simulink library "lib_Engine"  (R2017b)
settings: Solver=VariableStepAuto  StartTime=0.0  StopTime=10.0  RelTol=1e-3
undefined symbols (not defined in the file): air, Engine, env, max_vehicle_rad_air_flow
libraries: Pneumatic_lib x11, nesl_utility x9, simulink x5, EC2_libraries x1, fl_lib x1
settings Model: Creator=Di Russo  LastModifiedBy=Lyu19
settings CodeAppCC: StateflowObjectComments=on

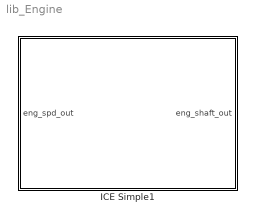
== system lib_Engine ==
  ICE Simple1 : Subsystem
      mask Display:
      | image(imread('EngineTopLevel.jpg'),'center')
      | color('red');
      | port_label('input',1,'SpdOut')
      | port_label('output',1,'ShaftOut')

== system lib_Engine/ICE Simple1 ==
  eng_spd_out : Inport
  Engine Plant Modified : Subsystem
      mask Display:
      | image(imread('EngineTopLevel.jpg'),'center')
      | color('red');
      | port_label('input',2,'SpdOut')
      | port_label('output',2,'ShaftOut')
  Inputs : Subsystem
  Soft ECM : Subsystem
      mask Display: image('SoftECU.jpg')
  eng_shaft_out : Outport
  tag scope: ECM_to_HCU=global
  wires:
  Engine Plant Modified/1(Out) -> Soft ECM/2(In1)
  Soft ECM/1(Out) -> [ECM_to_HCU]
  Inputs/1(Inputs) -> Soft ECM/1(In)
  Soft ECM/2(Out1) -> Engine Plant Modified/1("In ")  "ECM_to_Actuators"
  eng_spd_out/1 -> Engine Plant Modified/2(eng_spd_out)
  Engine Plant Modified/2(eng_shaft_out) -> eng_shaft_out/1

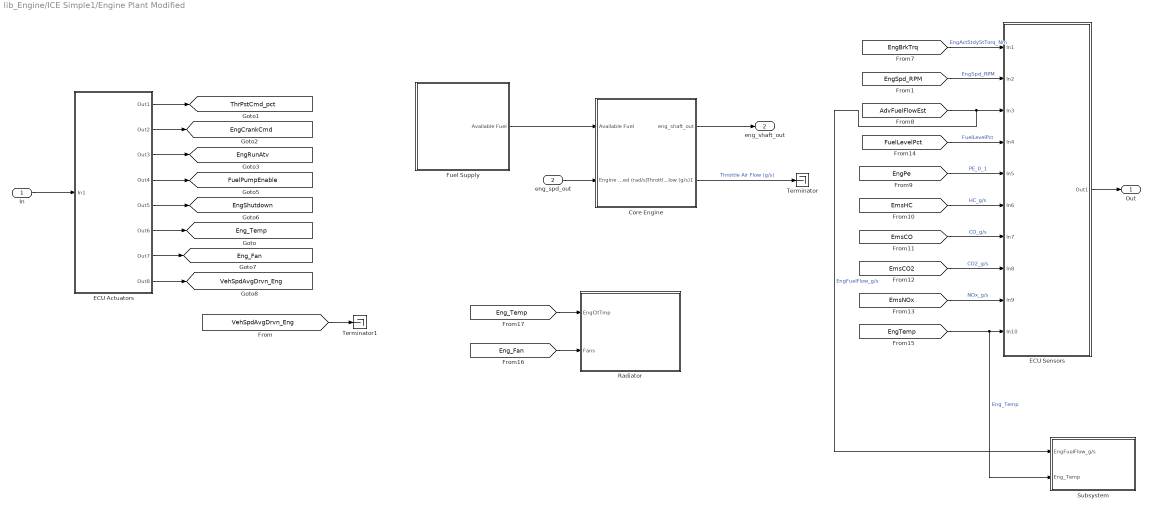
== system lib_Engine/ICE Simple1/Engine Plant Modified ==
  "In " : Inport
  eng_spd_out : Inport  Port=2
  Core Engine : Subsystem
      mask Display: image(imread('EngineShortBlock.jpg'),'center')
  ECU Actuators : Subsystem
  ECU Sensors : Subsystem
  Fuel Supply : Subsystem
      mask Display: image(imread('FuelTank.jpg'),'center')
  Radiator : Subsystem
  Subsystem : Subsystem
  Terminator : Terminator
  Terminator1 : Terminator
  Out : Outport
  eng_shaft_out : Outport  Port=2
  tag scope: EngCrankCmd=global, EngRunAtv=global, EngShutdown=global, Eng_Fan=global, Eng_Temp=global, FuelPumpEnable=global, ThrPstCmd_pct=global, VehSpdAvgDrvn_Eng=global
  wires:
  [VehSpdAvgDrvn_Eng] -> Terminator1/1
  Core Engine/2(Throttle Air Flow (g/s)1) -> Terminator/1  "Throttle Air Flow (g/s)"
  ECU Sensors/1(Out1) -> Out/1
  ECU Actuators/8(Out8) -> [VehSpdAvgDrvn_Eng]
  ECU Actuators/7(Out7) -> [Eng_Fan]
  ECU Actuators/6(Out6) -> [Eng_Temp]
  [Eng_Temp] -> Radiator/1(EngCltTmp)
  [Eng_Fan] -> Radiator/2(Fans)
  eng_spd_out/1 -> Core Engine/2(Engine Speed (rad/s))
  Core Engine/1(eng_shaft_out) -> eng_shaft_out/1
  ECU Actuators/3(Out3) -> [EngRunAtv]
  ECU Actuators/2(Out2) -> [EngCrankCmd]
  [EngSpd_RPM] -> ECU Sensors/2(In2)  "EngSpd_RPM"
  [EngBrkTrq] -> ECU Sensors/1(In1)  "EngActStdyStTorq_Nm"
  "In "/1 -> ECU Actuators/1(In1)
  ECU Actuators/1(Out1) -> [ThrPstCmd_pct]
  ECU Actuators/4(Out4) -> [FuelPumpEnable]
  Fuel Supply/1(Available Fuel) -> Core Engine/1(Available Fuel)
  [EmsNOx] -> ECU Sensors/9(In9)  "NOx_g/s"
  [EmsCO2] -> ECU Sensors/8(In8)  "CO2_g/s"
  [EmsCO] -> ECU Sensors/7(In7)  "CO_g/s"
  [EngPe] -> ECU Sensors/5(In5)  "PE_0_1"
  [EmsHC] -> ECU Sensors/6(In6)  "HC_g/s"
  [FuelLevelPct] -> ECU Sensors/4(In4)  "FuelLevelPct"
  ECU Actuators/5(Out5) -> [EngShutdown]
  [EngTemp] -> ECU Sensors/10(In10), Subsystem/2(Eng_Temp)  "Eng_Temp"
  [AdvFuelFlowEst] -> Subsystem/1(EngFuelFlow_g/s), ECU Sensors/3(In3)  "EngFuelFlow_g/s"

== system lib_Engine/ICE Simple1/Inputs ==
  Analog : Subsystem
  Bus Creator : BusCreator  Inputs=2
  CAN_from_HCU : Subsystem
  Inputs : Outport
  wires:
  Bus Creator/1 -> Inputs/1
  Analog/1(Out1) -> Bus Creator/2  "Analog"
  CAN_from_HCU/1(Out1) -> Bus Creator/1  "CAN"

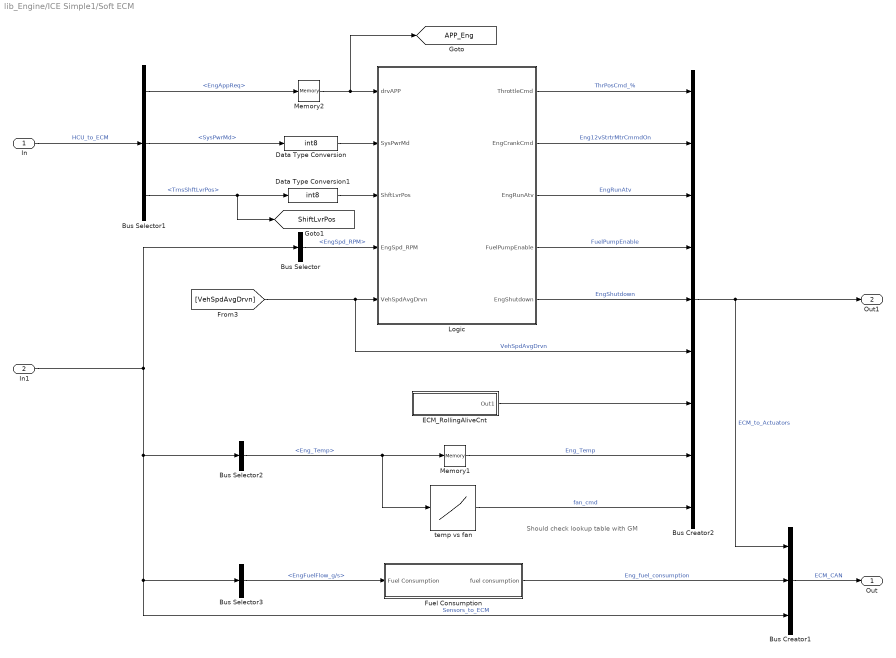
== system lib_Engine/ICE Simple1/Soft ECM ==
  note: Should check lookup table with GM
  In : Inport
  In1 : Inport  Port=2
  Bus Creator1 : BusCreator  Inputs=3
  Bus Creator2 : BusCreator  Inputs=9
  Bus Selector : BusSelector  OutputSignals=EngSpd_RPM
  Bus Selector1 : BusSelector  OutputSignals=Analog.EngAppReq,CAN.to EBCAN.PPEI_Platform_General_Status.SysPwrMd,CAN.to EBCAN.PPEI_Trans_General_Status_2.TrnsShftLvrPos
  Bus Selector2 : BusSelector  OutputSignals=Eng_Temp
  Bus Selector3 : BusSelector  OutputSignals=EngFuelFlow_g/s
  Data Type Conversion : DataTypeConversion  OutDataTypeStr=int8
  Data Type Conversion1 : DataTypeConversion  OutDataTypeStr=int8
  ECM_RollingAliveCnt : Subsystem
  Fuel Consumption : Subsystem
  Logic : Stateflow chart  TreatAsAtomicUnit=on
  Memory1 : Memory  InitialCondition=Engine.Init_T_amb
  Memory2 : Memory
  temp vs fan : Lookup_n-D  NumberOfTableDimensions=1  BreakpointsForDimension1=[0:1:100]  Table=[0:0.01:1]  InternalRulePriority=Speed  RndMeth=Simplest  InputSameDT=on
  Out : Outport
  Out1 : Outport  Port=2
  tag scope: APP_Eng=global, ShiftLvrPos=global
  wires:
  [VehSpdAvgDrvn] -> Logic/5(VehSpdAvgDrvn), Bus Creator2/6  "VehSpdAvgDrvn"
  In/1 -> Bus Selector1/1  "HCU_to_ECM"
  Memory2/1 -> Logic/1(drvAPP), [APP_Eng]
  Data Type Conversion1/1 -> Logic/3(ShftLvrPos)
  Data Type Conversion/1 -> Logic/2(SysPwrMd)
  ECM_RollingAliveCnt/1(Out1) -> Bus Creator2/7
  Memory1/1 -> Bus Creator2/8  "Eng_Temp"
  temp vs fan/1 -> Bus Creator2/9  "fan_cmd"
  Fuel Consumption/1(fuel consumption) -> Bus Creator1/2  "Eng_fuel_consumption"
  Bus Selector3/1 -> Fuel Consumption/1(Fuel Consumption)  "<EngFuelFlow_g/s>"
  Bus Selector2/1 -> Memory1/1, temp vs fan/1  "<Eng_Temp>"
  Logic/5(EngShutdown) -> Bus Creator2/5  "EngShutdown"
  Bus Selector1/3 -> Data Type Conversion1/1, [ShiftLvrPos]  "<TrnsShftLvrPos>"
  Bus Selector1/2 -> Data Type Conversion/1  "<SysPwrMd>"
  Logic/4(FuelPumpEnable) -> Bus Creator2/4  "FuelPumpEnable"
  In1/1 -> Bus Selector/1, Bus Selector2/1, Bus Selector3/1, Bus Creator1/3  "Sensors_to_ECM"
  Logic/1(ThrottleCmd) -> Bus Creator2/1  "ThrPosCmd_%"
  Bus Creator2/1 -> Bus Creator1/1, Out1/1  "ECM_to_Actuators"
  Bus Creator1/1 -> Out/1  "ECM_CAN"
  Logic/2(EngCrankCmd) -> Bus Creator2/2  "Eng12vStrtrMtrCmmdOn"
  Bus Selector1/1 -> Memory2/1  "<EngAppReq>"
  Bus Selector/1 -> Logic/4(EngSpd_RPM)  "<EngSpd_RPM>"
  Logic/3(EngRunAtv) -> Bus Creator2/3  "EngRunAtv"

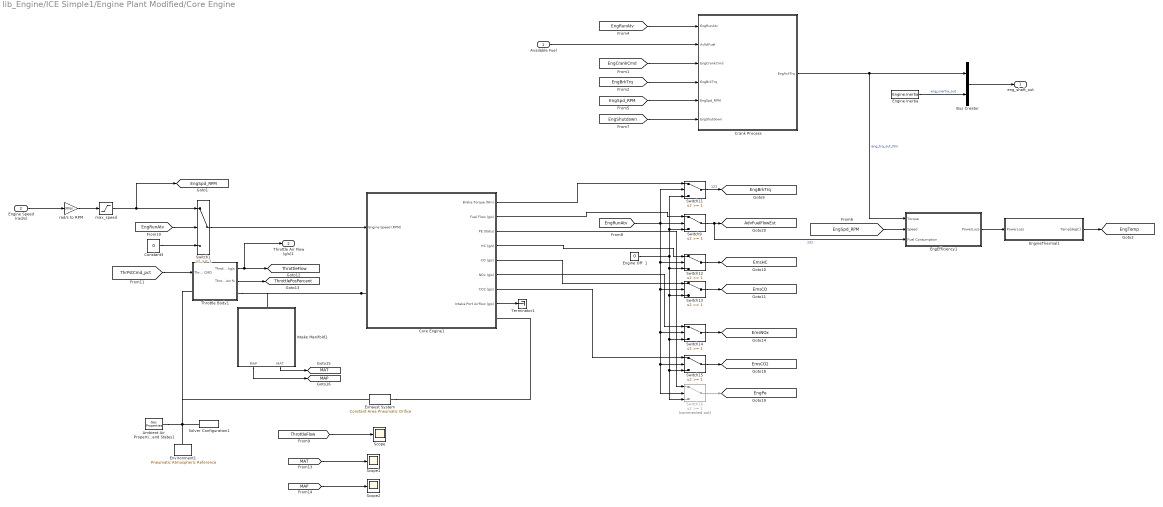
== system lib_Engine/ICE Simple1/Engine Plant Modified/Core Engine ==
  Available Fuel : Inport
  Engine Speed (rad/s) : Inport  Port=2
  Ambient Air Properties and States1 : Pneumatic_lib/Pneumatic Utilities/Gas Properties  c_p=1.005e+3 J/kg/K  c_v=717.95 J/kg/K  viscosity=1.821e-5 s*Pa  Pa=100 kPa  Ta=293.15 K  range_error=1
  Bus Creator : BusCreator  Inputs=2
  Constant3 : Constant  Value=0
  Core Engine1 : Subsystem
      mask Display: image(imread('EngineShortBlock.jpg'),'center')
  Crank Process : Stateflow chart  TreatAsAtomicUnit=on
  EngEfficiency1 : Subsystem
  Engine Inertia : Constant  Value=Engine.Inertia
  Engine Off  1 : Constant  Value=0
  EngineThermal1 : Subsystem
  Environment1 : Pneumatic_lib/Pneumatic Elements/Pneumatic Atmospheric Reference
  Exhaust System : Pneumatic_lib/Pneumatic Elements/Constant Area Pneumatic Orifice  Cd=0.8  Area=0.25*pi*(4*0.0254)^2 m^2  G_specify=off  G_priority=High  G=0 kg/s  G_nominal_specify=off  G_nominal_unit=kg/s  G_nominal_value=1  Q1_specify=off  Q1_priority=High  Q1=0 J/s  Q1_nominal_specify=off  Q1_nominal_unit=J/s  Q1_nominal_value=1  Q2_specify=off  Q2_priority=High  Q2=0 J/s  Q2_nominal_specify=off  Q2_nominal_unit=J/s  Q2_nominal_value=1  p1_specify=off  p1_priority=High  p1=1e+5 Pa  p1_nominal_specify=off  p1_nominal_unit=Pa  p1_nominal_value=1  p2_specify=off  p2_priority=High  p2=1e+5 Pa  p2_nominal_specify=off  p2_nominal_unit=Pa  p2_nominal_value=1  T1_specify=off  T1_priority=High  T1=300 K  T1_nominal_specify=off  T1_nominal_unit=K  T1_nominal_value=1  T2_specify=off  T2_priority=High  T2=300 K  T2_nominal_specify=off  T2_nominal_unit=K  T2_nominal_value=1
  Intake Manifold1 : Subsystem
      mask Display: image(imread('IntakeManifold.jpg'),'center')
  Scope : Scope
  Scope1 : Scope
  Scope2 : Scope
  Solver Configuration1 : nesl_utility/Solver Configuration  PhysicalDomain=network_engine_domain  SubClassName=solver  LeftPortType=input  RightPortType=generic  Accelerate=off  Tones=[]  Harmonics=[]  SimulateNoise=off  Profile=off  UseLocalSampling=off  EnableSwitchedLinearOptims=on  FrequencyDomain=off  UseCCode=off  RelTol=0.001  AbsTol=1e-06  MinStep=1e-09  ToWorkspace=off  RevertToSquareIcSolve=off  NumHomotopyIterations=100  PhasorMode=off  PhasorModeNumHarmonics=1  DoDC=off  ResidualTolerance=1e-9  UseLocalSolver=on  LocalSolverChoice=NE_BACKWARD_EULER_ADVANCER  LocalSolverSampleTime=.01  DoFixedCost=off  MaxNonlinIter=3  MaxModeIter=2  LinearAlgebra=Sparse  DelaysMemoryBudget=1024  AutomaticFiltering=on  FilteringTimeConstant=0.001
  Switch{1,9,11..15} (7 alike) : Switch  Threshold=1
  Switch16 : Switch  Commented=on  Threshold=1
  Terminator1 : Terminator
  Throttle Body1 : Subsystem
      mask Display: image(imread('ElectronicThrottle.jpg'),'center')
  max_speed : Saturate  UpperLimit=max(Engine.Engine.TQ.SPEED)  LowerLimit=0
  rad/s to RPM : Gain  Gain=30/pi
  eng_shaft_out : Outport
  Throttle Air Flow (g/s)1 : Outport  Port=2
  tag scope: AdvFuelFlowEst=global, EmsCO2=global, EmsCO=global, EmsHC=global, EmsNOx=global, EngBrkTrq=global, EngPe=global, EngSpd_RPM=global, EngTemp=global, MAP=global, MAT=global, ThrottleFlow=global, ThrottlePosPercent=global
  wires:
  Engine Speed (rad/s)/1 -> rad/s to RPM/1
  max_speed/1 -> Switch1/1, [EngSpd_RPM]
  rad/s to RPM/1 -> max_speed/1
  [MAP] -> Scope2/1
  [MAT] -> Scope1/1
  [ThrottleFlow] -> Scope/1
  [EngBrkTrq] -> Crank Process/4(EngBrkTrq)
  [EngShutdown] -> Crank Process/6(EngShutdown)
  [EngRunAtv] -> Crank Process/1(EngRunAtv)
  Bus Creator/1 -> eng_shaft_out/1
  Available Fuel/1 -> Crank Process/2(AvlblFuel)
  [EngCrankCmd] -> Crank Process/3(EngCrankCmd)
  [EngSpd_RPM] -> Crank Process/5(EngSpd_RPM)
  Engine Inertia/1 -> Bus Creator/2  "eng_inertia_out"
  Engine Off  1/1 -> Switch12/3, Switch13/3, Switch14/3, Switch15/3, Switch16/3, Switch11/3, Switch9/3
  Core Engine1/5(CO (g/s)) -> Switch13/1
  Core Engine1/2(Fuel Flow (g/s)) -> Switch9/1
  Core Engine1/7(CO2 (g/s)) -> Switch15/1
  Switch12/1 -> [EmsHC]
  Switch11/1 -> [EngBrkTrq]  "123"
  Switch15/1 -> [EmsCO2]
  Switch9/1 -> EngEfficiency1/3(Fuel Consumption), [AdvFuelFlowEst]  "131"
  [EngSpd_RPM] -> EngEfficiency1/2(Speed)
  Switch13/1 -> [EmsCO]
  EngineThermal1/1(Temp[degC]) -> [EngTemp]
  Core Engine1/6(NOx (g/s)) -> Switch14/1
  Switch14/1 -> [EmsNOx]
  [EngRunAtv] -> Switch9/2, Switch12/2, Switch15/2, Switch16/2, Switch14/2, Switch13/2, Switch11/2
  EngEfficiency1/1(PowerLoss) -> EngineThermal1/1(PowerLoss)
  Crank Process/1(EngActTrq) -> Bus Creator/1, EngEfficiency1/1(Torque)  "eng_trq_out_Nm"
  Switch16/1 -> [EngPe]
  Core Engine1/1(Brake Torque (Nm)) -> Switch11/1
  Core Engine1/4(HC (g/s)) -> Switch12/1
  Core Engine1/3(PE Status) -> Switch16/1
  [ThrPstCmd_pct] -> Throttle Body1/1(Throttle Position % CMD)
  Switch1/1 -> Core Engine1/1(Engine Speed (RPM))
  Constant3/1 -> Switch1/3
  [EngRunAtv] -> Switch1/2
  Throttle Body1/1(Throttle Flow kg/s) -> [ThrottleFlow], Throttle Air Flow (g/s)1/1
  Intake Manifold1/2(MAT) -> [MAT]
  Intake Manifold1/1(MAP) -> [MAP]
  Core Engine1/8(Intake Port Airflow (g/s)) -> Terminator1/1
  Throttle Body1/2(Throttle Position %) -> [ThrottlePosPercent]
  connections:
  Exhaust System/LConn1 -- Core Engine1/RConn1
  Core Engine1/LConn1 -- Intake Manifold1/LConn1 -- Throttle Body1/RConn1
  Ambient Air Properties and States1/RConn1 -- Throttle Body1/LConn1 -- Exhaust System/RConn1 -- Solver Configuration1/RConn1 -- Environment1/LConn1

== system lib_Engine/ICE Simple1/Engine Plant Modified/ECU Actuators ==
  In1 : Inport
  Bus Selector : BusSelector  OutputSignals=ThrPosCmd_%,Eng12vStrtrMtrCmmdOn,EngRunAtv,FuelPumpEnable,EngShutdown,Eng_Temp,fan_cmd,VehSpdAvgDrvn
  Out1 : Outport
  Out2 : Outport  Port=2
  Out3 : Outport  Port=3
  Out4 : Outport  Port=4
  Out5 : Outport  Port=5
  Out6 : Outport  Port=6
  Out7 : Outport  Port=7
  Out8 : Outport  Port=8
  wires:
  Bus Selector/8 -> Out8/1  "<VehSpdAvgDrvn>"
  Bus Selector/7 -> Out7/1  "<fan_cmd>"
  Bus Selector/6 -> Out6/1  "<Eng_Temp>"
  Bus Selector/3 -> Out3/1  "<EngRunAtv>"
  Bus Selector/2 -> Out2/1  "<Eng12vStrtrMtrCmmdOn>"
  Bus Selector/1 -> Out1/1  "<ThrPosCmd_%>"
  In1/1 -> Bus Selector/1
  Bus Selector/4 -> Out4/1  "<FuelPumpEnable>"
  Bus Selector/5 -> Out5/1  "<EngShutdown>"

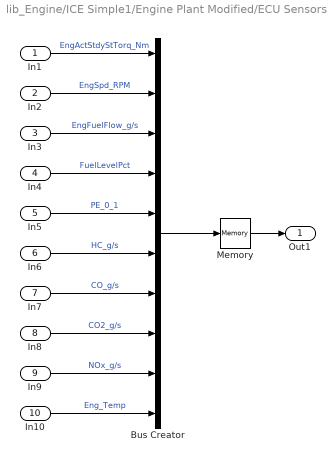
== system lib_Engine/ICE Simple1/Engine Plant Modified/ECU Sensors ==
  In1 : Inport
  In2 : Inport  Port=2
  In3 : Inport  Port=3
  In4 : Inport  Port=4
  In5 : Inport  Port=5
  In6 : Inport  Port=6
  In7 : Inport  Port=7
  In8 : Inport  Port=8
  In9 : Inport  Port=9
  In10 : Inport  Port=10
  Bus Creator : BusCreator  Inputs=10
  Memory : Memory
  Out1 : Outport
  wires:
  Memory/1 -> Out1/1
  In10/1 -> Bus Creator/10  "Eng_Temp"
  In8/1 -> Bus Creator/8  "CO2_g/s"
  Bus Creator/1 -> Memory/1
  In7/1 -> Bus Creator/7  "CO_g/s"
  In6/1 -> Bus Creator/6  "HC_g/s"
  In5/1 -> Bus Creator/5  "PE_0_1"
  In4/1 -> Bus Creator/4  "FuelLevelPct"
  In3/1 -> Bus Creator/3  "EngFuelFlow_g/s"
  In2/1 -> Bus Creator/2  "EngSpd_RPM"
  In1/1 -> Bus Creator/1  "EngActStdyStTorq_Nm"
  In9/1 -> Bus Creator/9  "NOx_g/s"

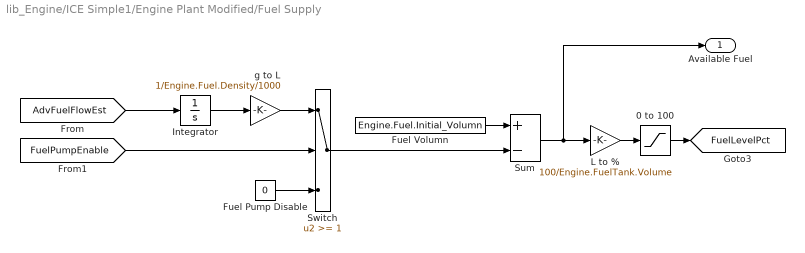
== system lib_Engine/ICE Simple1/Engine Plant Modified/Fuel Supply ==
  0 to 100 : Saturate
  Fuel Pump Disable : Constant  Value=0
  Fuel Volumn : Constant  Value=Engine.Fuel.Initial_Volumn
  Integrator : Integrator  LimitOutput=on  UpperSaturationLimit=Engine.FuelTank.Volume  LowerSaturationLimit=0
  L to % : Gain  Gain=100/Engine.FuelTank.Volume
  Sum : Sum  Inputs=+-
  Switch : Switch  Threshold=1
  g to L : Gain  Gain=1/Engine.Fuel.Density/1000
  Available Fuel : Outport
  tag scope: FuelLevelPct=global
  wires:
  Fuel Volumn/1 -> Sum/1
  Switch/1 -> Sum/2
  Sum/1 -> Available Fuel/1, L to %/1
  [FuelPumpEnable] -> Switch/2
  [AdvFuelFlowEst] -> Integrator/1
  Integrator/1 -> g to L/1
  g to L/1 -> Switch/1
  Fuel Pump Disable/1 -> Switch/3
  L to %/1 -> 0 to 100/1
  0 to 100/1 -> [FuelLevelPct]

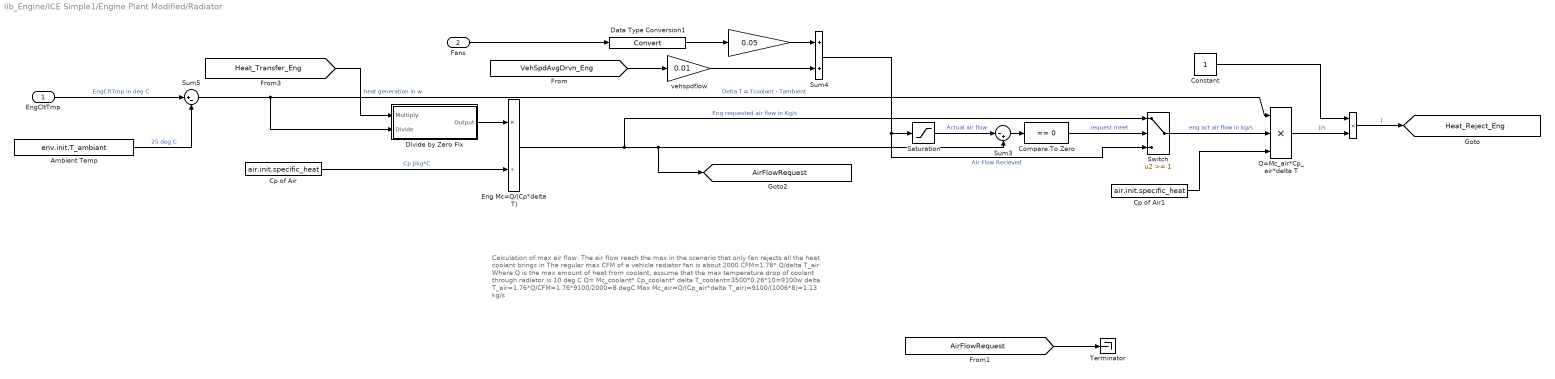
== system lib_Engine/ICE Simple1/Engine Plant Modified/Radiator ==
  note: Calculation of max air flow:
      |
      | The air flow reach the max in the scenario that only fan rejects all the heat coolant brings in
      |
      | The regular max CFM of a vehicle radiator fan is about 2000
      |
      | CFM=1.76* Q/delta T_air
      |
      | Where Q is the max amount of heat from coolant, assume that the max temperature drop of coolant
      | through radiator is 10 deg C
      |
      | Q= Mc_coolant* Cp_coolant* delta T_coolant=3500*0.26*10=9100w
      |
      | delta T_air=1.76*Q/CFM=1.76*9100/2000=8 degC
      |
      | Max Mc_air=Q/(Cp_air*delta T_air)=9100/(1006*8)=1.13 kg/s
  EngCltTmp : Inport
  Fans : Inport  Port=2
  " " : Product  Inputs=**
  " " : Gain  Gain=0.05
  Ambient Temp : Constant  Value=env.init.T_ambiant
  Compare To Zero : simulink/Logic and Bit Operations/Compare To Zero  relop===  OutDataTypeStr=uint8
  Constant : Constant
  Cp of Air : Constant  Value=air.init.specific_heat
  Cp of Air1 : Constant  Value=air.init.specific_heat
  Data Type Conversion1 : DataTypeConversion
  Divide by Zero Fix : Subsystem
  "Eng Mc=Q/(Cp*delta T) " : Product  Inputs=*/
  Q=Mc_air*Cp_air*delta T : Product  Inputs=***
  Saturation : Saturate  UpperLimit=max_vehicle_rad_air_flow  LowerLimit=-1
  Sum3 : Sum  Inputs=|-+
  Sum4 : Sum
  Sum5 : Sum  Inputs=|+-
  Switch : Switch  Threshold=1
  Terminator : Terminator
  vehspdflow : Gain  Gain=0.01
  tag scope: AirFlowRequest=global, Heat_Reject_Eng=global
  wires:
  [AirFlowRequest] -> Terminator/1
  Constant/1 -> " "/1
  " "/1 -> Sum4/1
  Divide by Zero Fix/1(Output) -> "Eng Mc=Q/(Cp*delta T) "/1
  [Heat_Transfer_Eng] -> Divide by Zero Fix/1(Multiply)  "heat generation in w"
  vehspdflow/1 -> Sum4/2
  [VehSpdAvgDrvn_Eng] -> vehspdflow/1
  Fans/1 -> Data Type Conversion1/1
  Sum4/1 -> Saturation/1, Switch/3  "Air Flow Recieved"
  "Eng Mc=Q/(Cp*delta T) "/1 -> [AirFlowRequest], Sum3/2, Switch/1  "Eng requested air flow in Kg/s"
  EngCltTmp/1 -> Sum5/1  "EngCltTmp in deg C"
  Sum5/1 -> Q=Mc_air*Cp_air*delta T/1, Divide by Zero Fix/2(Divide)  "Delta T = Tcoolant - Tambient"
  Ambient Temp/1 -> Sum5/2  "25 deg C"
  Cp of Air/1 -> "Eng Mc=Q/(Cp*delta T) "/2  "Cp J/kg*C"
  Compare To Zero/1 -> Switch/2  "request meet"
  Sum3/1 -> Compare To Zero/1
  Saturation/1 -> Sum3/1  "Actual air flow"
  " "/1 -> [Heat_Reject_Eng]  "J"
  Q=Mc_air*Cp_air*delta T/1 -> " "/2  "J/s"
  Switch/1 -> Q=Mc_air*Cp_air*delta T/2  "eng act air flow in kg/s"
  Cp of Air1/1 -> Q=Mc_air*Cp_air*delta T/3
  Data Type Conversion1/1 -> " "/1

== system lib_Engine/ICE Simple1/Engine Plant Modified/Subsystem ==
  EngFuelFlow_g/s : Inport
  Eng_Temp : Inport  Port=2
  Rate Transition1 : RateTransition  OutPortSampleTime=1
  Rate Transition7 : RateTransition  OutPortSampleTime=1
  To Workspace2 : ToWorkspace  VariableName=EngCltTmp  SampleTime=-1
  To Workspace3 : ToWorkspace  VariableName=InstFuelConsmpRate  SampleTime=-1
  g/s 2 l/hr : Gain  Gain=0.001/0.7871*3600
  wires:
  EngFuelFlow_g/s/1 -> g/s 2 l/hr/1
  Eng_Temp/1 -> Rate Transition1/1
  Rate Transition1/1 -> To Workspace2/1
  g/s 2 l/hr/1 -> Rate Transition7/1
  Rate Transition7/1 -> To Workspace3/1

== system lib_Engine/ICE Simple1/Inputs/Analog ==
  Out1 : Outport
  wires:
  [Analog] -> Out1/1

== system lib_Engine/ICE Simple1/Inputs/CAN_from_HCU ==
  Bus Creator : BusCreator  Inputs=2
  Out1 : Outport
  wires:
  Bus Creator/1 -> Out1/1
  [HCU_to_VEH_CAN] -> Bus Creator/2
  [HCU_to_EBCAN] -> Bus Creator/1

== system lib_Engine/ICE Simple1/Soft ECM/ECM_RollingAliveCnt ==
  Constant : Constant
  Constant1 : Constant  Value=0
  Rolling Alive Counter : Stateflow chart  TreatAsAtomicUnit=on
  Switch : Switch  Criteria=u2 > Threshold
  Out1 : Outport
  tag scope: ECM_CAN_fault=global
  wires:
  Constant1/1 -> [ECM_CAN_fault]
  Switch/1 -> Out1/1  "ECM_RollingAliveCnt"
  Rolling Alive Counter/1(RollingAliveCnt) -> Switch/3
  Constant/1 -> Switch/1
  [ECM_CAN_fault] -> Switch/2

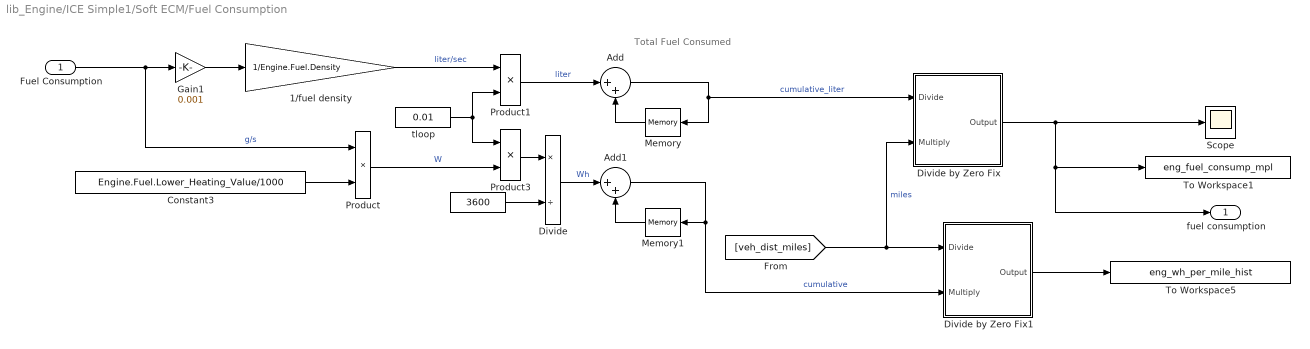
== system lib_Engine/ICE Simple1/Soft ECM/Fuel Consumption ==
  note: Total Fuel Consumed
  Fuel Consumption : Inport
  " " : Constant  Value=3600
  " tloop" : Constant  Value=0.01
  1/fuel density : Gain  Gain=1/Engine.Fuel.Density
  Add : Sum  Inputs=|++
  Add1 : Sum  Inputs=|++
  Constant3 : Constant  Value=Engine.Fuel.Lower_Heating_Value/1000
  Divide : Product  Inputs=*/
  Divide by Zero Fix : Subsystem
  Divide by Zero Fix1 : Subsystem
  Gain1 : Gain  Gain=0.001
  Memory : Memory
  Memory1 : Memory
  Product : Product  RndMeth=Zero
  Product1 : Product  RndMeth=Zero
  Product3 : Product  RndMeth=Zero
  Scope : Scope
  To Workspace1 : ToWorkspace  VariableName=eng_fuel_consump_mpl  SampleTime=-1
      settings: Decimation=WORKSPACE_DECIMATION
  To Workspace5 : ToWorkspace  VariableName=eng_wh_per_mile_hist  SampleTime=-1
      settings: Decimation=WORKSPACE_DECIMATION
  fuel consumption : Outport
  wires:
  Gain1/1 -> 1/fuel density/1
  " "/1 -> Divide/2
  Product3/1 -> Divide/1
  " tloop"/1 -> Product1/2, Product3/1
  Add/1 -> Memory/1, Divide by Zero Fix/1(Divide)  "cumulative_liter"
  Memory/1 -> Add/2
  Fuel Consumption/1 -> Gain1/1, Product/1  "g/s"
  1/fuel density/1 -> Product1/1  "liter/sec"
  Product1/1 -> Add/1  "liter"
  [veh_dist_miles] -> Divide by Zero Fix/2(Multiply), Divide by Zero Fix1/1(Divide)  "miles"
  Divide by Zero Fix/1(Output) -> Scope/1, To Workspace1/1, fuel consumption/1
  Constant3/1 -> Product/2
  Product/1 -> Product3/2  "W"
  Add1/1 -> Memory1/1, Divide by Zero Fix1/2(Multiply)  "cumulative"
  Memory1/1 -> Add1/2
  Divide/1 -> Add1/1  "Wh"
  Divide by Zero Fix1/1(Output) -> To Workspace5/1

== system lib_Engine/ICE Simple1/Soft ECM/Logic/APP2TP ==
  APP : Inport
  EngSpd : Inport  Port=2
  f : TriggerPort  TriggerType=function-call  VariantControl=Variant
      settings: CopyFcn=Stateflow.SLINSF.SimulinkMan.removeBlockPreDeleteFcn  PreDeleteFcn=Stateflow.SLINSF.SimulinkMan.unsafePredeleteFcn
  Based on APP to TP test data from 2013 Malibu1 : Lookup_n-D  NumberOfTableDimensions=1  BreakpointsForDimension1=[0,1,2,3,4,5,6,7,8,9,10,11,12,13,14,15,16,17,18,19,20,21,22,23,24,25,26,27,28,29,30,31,32,33,34,35,36,37,38,39,40,41,42,43,44,45,46,48,51,55,60,66,100]  Table=[0,6.3,12.7686537241448,12.6326703204763,12.8888951657611,13.4307541011932,14.1739282202018,15.0532596030224,16.0198646102832,17.0384547356068,18.0848650172271,19.1437900086214,20.206727308158,21.2701286477589,22.3337585405773,23.3992604876916,24.4689307438132,25.5446996420107,26.6273204774486,27.7157659501418,28.8068321667249,29.8949502012373,30.9722052149229,32.0285631350456,33.0523048927199,34.0306682197568,34.9506970045247,35.8002982068255,36.5695063317874,37.2519554627699,37.846558853288,38.359396077948,38.8058077424007,39.2126977523099,39.6210431413345,40.0886114581279,40.6928857123509,41.5341968797017,42.7390639659588,44.4637416300428,46.8979753660875,50.2689642445339,54.8455312122302,60.9425009515619,68.9252852985734,79.2146762201353,81.9427,84.6943,87.2166,89.5096,91.3439,92.6051,100]  ExtrapMethod=Clip  UseLastTableValue=on  InternalRulePriority=Speed  RndMeth=Simplest  InputSameDT=on
  Based on APP to TP test data from 2013 Malibu2 : Lookup_n-D  Commented=on  NumberOfTableDimensions=1  BreakpointsForDimension1=[0,1,2,3,4,5,6,7,8,9,10,11,12,13,14,15,16,17,18,19,20,21,22,23,24,25,26,27,28,29,30,31,32,33,34,35,36,37,38,39,40,41,42,43,44,45,46,48,51,55,60,66,100]  Table=[0,7,12.5,16,16.5,17,18,19,21,23,25,28,29,30,32,35,37,39,41,44,47,48,48.6,49,50,51.5,52,53,53.25,53.5,55,56.75,57,58,60,64,68,72,73,74,75,76,77,77.5,78,80,82,85,87,89.5,91.5,93,100]  ExtrapMethod=Clip  UseLastTableValue=on  InternalRulePriority=Speed  RndMeth=Simplest  InputSameDT=on
  Display : Display
  Product : Product
  RPM Derating : Lookup_n-D  NumberOfTableDimensions=1  BreakpointsForDimension1=[0 1000 2000 3000 4000 5000 6000 7000]  Table=[1 1 1 1 1 1 1 0]  ExtrapMethod=Clip  UseLastTableValue=on  InternalRulePriority=Speed  RndMeth=Simplest  InputSameDT=on
  Saturation : Saturate  UpperLimit=100  LowerLimit=0
  TP : Outport
  wires:
  Saturation/1 -> Product/1
  Based on APP to TP test data from 2013 Malibu1/1 -> Saturation/1  "1"
  APP/1 -> Display/1, Based on APP to TP test data from 2013 Malibu1/1  "3"
  RPM Derating/1 -> Product/2  "2"
  EngSpd/1 -> RPM Derating/1
  Product/1 -> TP/1

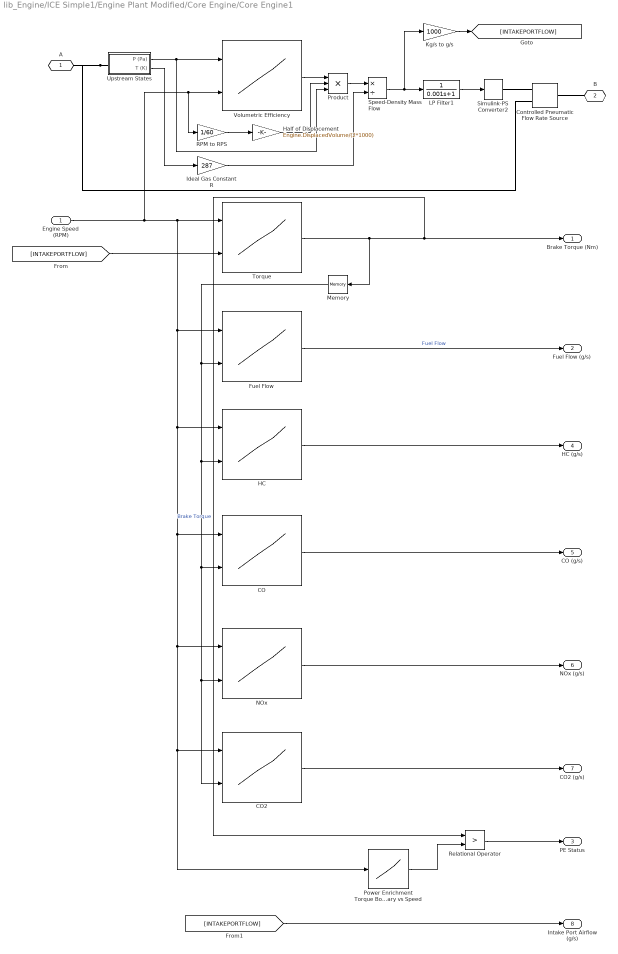
== system lib_Engine/ICE Simple1/Engine Plant Modified/Core Engine/Core Engine1 ==
  Engine Speed (RPM) : Inport
  CO : Lookup2D  RowIndex=Engine.Engine.Emissions.SPEED  ColumnIndex=Engine.Engine.Emissions.TQ  Table=Engine.Engine.Emissions.CO/1000  LookUpMeth=Interpolation-Use End Values
  CO2 : Lookup2D  RowIndex=Engine.Engine.Emissions.SPEED  ColumnIndex=Engine.Engine.Emissions.TQ  Table=Engine.Engine.Emissions.CO2/1000  LookUpMeth=Interpolation-Use End Values
  Controlled Pneumatic Flow Rate Source : Pneumatic_lib/Pneumatic Sources/Controlled Pneumatic Flow Rate Source
  Fuel Flow : Lookup2D  RowIndex=Engine.Engine.FuelFlow.SPEED  ColumnIndex=Engine.Engine.FuelFlow.TQ  Table=Engine.Engine.FuelFlow.FuelFlow  LookUpMeth=Interpolation-Use End Values
  HC : Lookup2D  RowIndex=Engine.Engine.Emissions.SPEED  ColumnIndex=Engine.Engine.Emissions.TQ  Table=Engine.Engine.Emissions.HC/1000  LookUpMeth=Interpolation-Use End Values
  Half of Displacement : Gain  Gain=Engine.DisplacedVolume/(2*1000)
  Ideal Gas Constant R : Gain  Gain=287
  Kg/s to g/s : Gain  Gain=1000
  LP Filter1 : TransferFcn  Denominator=[0.001 1]
  Memory : Memory
  NOx : Lookup2D  RowIndex=Engine.Engine.Emissions.SPEED  ColumnIndex=Engine.Engine.Emissions.TQ  Table=Engine.Engine.Emissions.NOx/1000  LookUpMeth=Interpolation-Use End Values
  Power Enrichment Torque Boundary vs Speed : Lookup_n-D  NumberOfTableDimensions=1  BreakpointsForDimension1=Engine.Engine.PEBound.SPEED  Table=Engine.Engine.PEBound.PEBound  ExtrapMethod=Clip  InternalRulePriority=Speed  RndMeth=Simplest  InputSameDT=on
  Product : Product  Inputs=***
  RPM to RPS : Gain  Gain=1/60
  Relational Operator : RelationalOperator  Operator=>  OutDataTypeStr=boolean  RndMeth=Nearest
  Simulink-PS Converter2 : nesl_utility/Simulink-PS Converter  PhysicalDomain=network_engine_domain  SubClassName=ps_input  LeftPortType=input  RightPortType=output  PseudoPeriodic=off  Frequencies=[]  NoiseDistribution=none  NoiseParameters=[]  Unit=kg/s  AffineConversion=off  FilteringAndDerivatives=zero  SimscapeFilterOrder=1  InputFilterTimeConstant=.001  UdotUserProvided=0
  Speed-Density Mass Flow : Product  Inputs=*/
  Torque : Lookup2D  RowIndex=Engine.Engine.TQ.SPEED  ColumnIndex=Engine.Engine.TQ.MAF  Table=Engine.Engine.TQ.TQ  LookUpMeth=Interpolation-Use End Values
  Upstream States : Subsystem
  Volumetric Efficiency : Lookup2D  RowIndex=Engine.Engine.VE.MAP  ColumnIndex=Engine.Engine.VE.SPEED  Table=Engine.Engine.VE.VE  LookUpMeth=Interpolation-Use End Values
  A : PMIOPort  Port=1  Side=Left
  B : PMIOPort  Port=2  Side=Right
  Brake Torque (Nm) : Outport
  Fuel Flow (g/s) : Outport  Port=2
  PE Status : Outport  Port=3
  HC (g/s) : Outport  Port=4
  CO (g/s) : Outport  Port=5
  NOx (g/s) : Outport  Port=6
  CO2 (g/s) : Outport  Port=7
  Intake Port Airflow (g/s) : Outport  Port=8
  wires:
  LP Filter1/1 -> Simulink-PS Converter2/1
  Speed-Density Mass Flow/1 -> Kg/s to g/s/1, LP Filter1/1
  [INTAKEPORTFLOW] -> Intake Port Airflow (g/s)/1
  CO2/1 -> CO2 (g/s)/1
  NOx/1 -> NOx (g/s)/1
  CO/1 -> CO (g/s)/1
  HC/1 -> HC (g/s)/1
  Relational Operator/1 -> PE Status/1
  Power Enrichment Torque Boundary vs Speed/1 -> Relational Operator/2
  Memory/1 -> Fuel Flow/2, HC/2, CO/2, NOx/2, CO2/2
  Engine Speed (RPM)/1 -> RPM to RPS/1, Volumetric Efficiency/2, CO2/1, Power Enrichment Torque Boundary vs Speed/1, NOx/1, CO/1, HC/1, Fuel Flow/1, Torque/1
  Fuel Flow/1 -> Fuel Flow (g/s)/1  "Fuel Flow"
  [INTAKEPORTFLOW] -> Torque/2
  Torque/1 -> Memory/1, Relational Operator/1, Brake Torque (Nm)/1  "Brake Torque"
  Kg/s to g/s/1 -> [INTAKEPORTFLOW]
  Half of Displacement/1 -> Product/2
  RPM to RPS/1 -> Half of Displacement/1
  Upstream States/2(T (K)) -> Ideal Gas Constant R/1
  Product/1 -> Speed-Density Mass Flow/1
  Ideal Gas Constant R/1 -> Speed-Density Mass Flow/2
  Volumetric Efficiency/1 -> Product/1
  Upstream States/1(P (Pa)) -> Product/3, Volumetric Efficiency/1
  connections:
  B/RConn1 -- Controlled Pneumatic Flow Rate Source/LConn1
  Simulink-PS Converter2/RConn1 -- Controlled Pneumatic Flow Rate Source/RConn2
  Upstream States/LConn1 -- Controlled Pneumatic Flow Rate Source/RConn1 -- A/RConn1

== system lib_Engine/ICE Simple1/Engine Plant Modified/Core Engine/Crank Process/function ==
  EngSpd : Inport
  f : TriggerPort  TriggerType=function-call  VariantControl=Variant
      settings: CopyFcn=Stateflow.SLINSF.SimulinkMan.removeBlockPreDeleteFcn  PreDeleteFcn=Stateflow.SLINSF.SimulinkMan.unsafePredeleteFcn
  1-D Lookup Table : Lookup_n-D  NumberOfTableDimensions=1  BreakpointsForDimension1=[0 50 120 210 300 320 340 350 400]  Table="[90 90 90 10 5 5  5 5 5]"  InternalRulePriority=Speed  RndMeth=Simplest  InputSameDT=on
  CrankTrq : Outport
  wires:
  1-D Lookup Table/1 -> CrankTrq/1
  EngSpd/1 -> 1-D Lookup Table/1

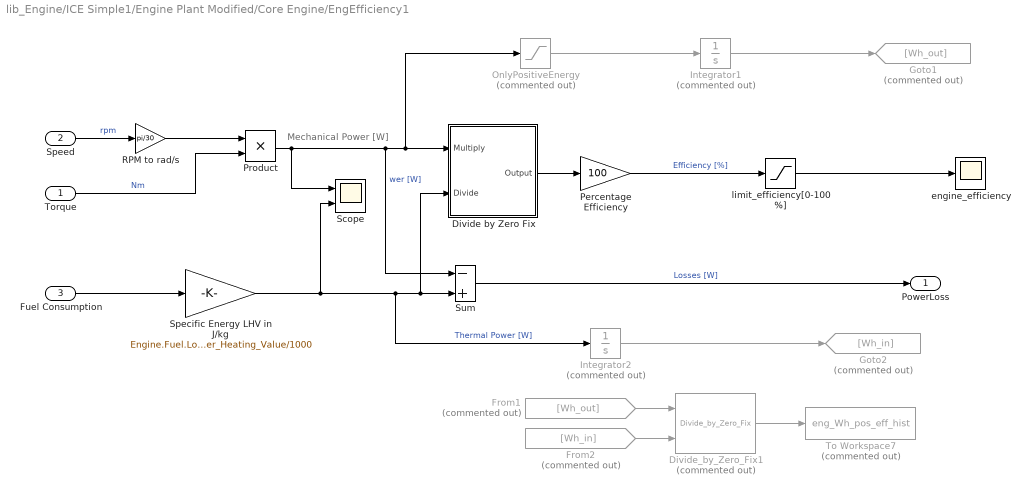
== system lib_Engine/ICE Simple1/Engine Plant Modified/Core Engine/EngEfficiency1 ==
  note: Mechanical Power [W]
  Torque : Inport
  Speed : Inport  Port=2
  Fuel Consumption : Inport  Port=3
  Divide by Zero Fix : Subsystem
  Divide_by_Zero_Fix1 : EC2_libraries/Divide_by_Zero_Fix  Commented=on
  From1 : From  Commented=on  GotoTag=Wh_out
  From2 : From  Commented=on  GotoTag=Wh_in
  Goto1 : Goto  Commented=on  GotoTag=Wh_out
  Goto2 : Goto  Commented=on  GotoTag=Wh_in
  Integrator1 : Integrator  Commented=on  LimitOutput=on  LowerSaturationLimit=0
  Integrator2 : Integrator  Commented=on  LimitOutput=on  LowerSaturationLimit=0
  OnlyPositiveEnergy : Saturate  Commented=on  UpperLimit=inf  LowerLimit=0
  Percentage Efficiency : Gain  Gain=100
  Product : Product  RndMeth=Zero
  "RPM to rad/s " : Gain  Gain=pi/30
  Scope : Scope  NumInputPorts=2
  Specific Energy LHV in J/kg : Gain  Gain=Engine.Fuel.Lower_Heating_Value/1000
  Sum : Sum  Inputs=-+
  To Workspace7 : ToWorkspace  Commented=on  VariableName=eng_Wh_pos_eff_hist  SampleTime=-1
      settings: Decimation=WORKSPACE_DECIMATION
  engine_efficiency : Scope
  limit_efficiency[0-100%] : Saturate  UpperLimit=100  LowerLimit=0
  PowerLoss : Outport
  wires:
  "RPM to rad/s "/1 -> Product/1
  Integrator2/1 -> Goto2/1
  OnlyPositiveEnergy/1 -> Integrator1/1
  Integrator1/1 -> Goto1/1
  From2/1 -> Divide_by_Zero_Fix1/2
  From1/1 -> Divide_by_Zero_Fix1/1
  Divide_by_Zero_Fix1/1 -> To Workspace7/1
  Product/1 -> Sum/1, OnlyPositiveEnergy/1, Divide by Zero Fix/1(Multiply), Scope/1  "wer [W]"
  Divide by Zero Fix/1(Output) -> Percentage Efficiency/1
  Percentage Efficiency/1 -> limit_efficiency[0-100%]/1  "Efficiency [%]"
  Speed/1 -> "RPM to rad/s "/1  "rpm"
  Torque/1 -> Product/2  "Nm"
  Specific Energy LHV in J/kg/1 -> Scope/2, Integrator2/1, Sum/2, Divide by Zero Fix/2(Divide)  "Thermal Power [W]"
  Fuel Consumption/1 -> Specific Energy LHV in J/kg/1
  Sum/1 -> PowerLoss/1  "Losses [W]"
  limit_efficiency[0-100%]/1 -> engine_efficiency/1

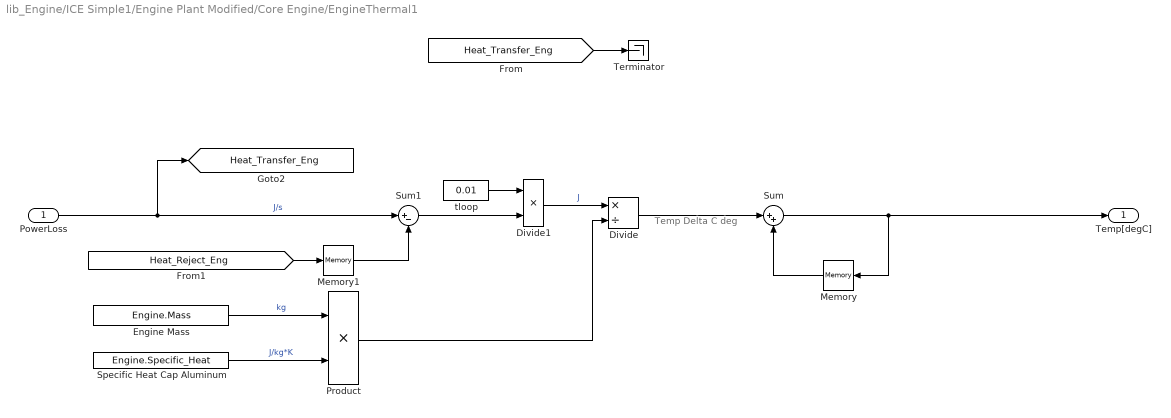
== system lib_Engine/ICE Simple1/Engine Plant Modified/Core Engine/EngineThermal1 ==
  note: Temp Delta C deg
  PowerLoss : Inport
  Divide : Product  Inputs=*/
  Divide1 : Product  Inputs=**
  Engine Mass : Constant  Value=Engine.Mass
  Memory : Memory  InitialCondition=Engine.Init_T_amb
  Memory1 : Memory
  Product : Product  RndMeth=Zero
  Specific Heat Cap Aluminum : Constant  Value=Engine.Specific_Heat
  Sum : Sum  Inputs=|++
  Sum1 : Sum  Inputs=|+-
  Terminator : Terminator
  tloop : Constant  Value=0.01
  Temp[degC] : Outport
  tag scope: Heat_Transfer_Eng=global
  wires:
  [Heat_Transfer_Eng] -> Terminator/1
  [Heat_Reject_Eng] -> Memory1/1
  tloop/1 -> Divide1/1
  Divide/1 -> Sum/1
  Sum/1 -> Temp[degC]/1, Memory/1
  Product/1 -> Divide/2
  Specific Heat Cap Aluminum/1 -> Product/2  "J/kg*K"
  Engine Mass/1 -> Product/1  "kg"
  PowerLoss/1 -> [Heat_Transfer_Eng], Sum1/1  "J/s"
  Memory/1 -> Sum/2
  Sum1/1 -> Divide1/2
  Divide1/1 -> Divide/1  "J"
  Memory1/1 -> Sum1/2

== system lib_Engine/ICE Simple1/Engine Plant Modified/Core Engine/Intake Manifold1 ==
  Heat-Transfer Neglected : fl_lib/Thermal/Thermal Elements/Perfect Insulator  T_specify=off  T_priority=None  T=0 K  T_nominal_specify=off  T_nominal_unit=K  T_nominal_value=1
      settings: SourceProductName=Simscape
  Intake Manifold Volume1 : Pneumatic_lib/Pneumatic Elements/Constant Volume Pneumatic Chamber  Volume=Engine.IntakeManifold.Volume l  pressure_specify=on  pressure_priority=High  pressure=26 kPa  pressure_nominal_specify=off  pressure_nominal_unit=Pa  pressure_nominal_value=1  temperature_specify=on  temperature_priority=High  temperature=20 K  temperature_nominal_specify=off  temperature_nominal_unit=K  temperature_nominal_value=1  gas_flow_specify=off  gas_flow_priority=High  gas_flow=0 kg/s  gas_flow_nominal_specify=off  gas_flow_nominal_unit=kg/s  gas_flow_nominal_value=1  heat_flow_specify=off  heat_flow_priority=High  heat_flow=0 J/s  heat_flow_nominal_specify=off  heat_flow_nominal_unit=J/s  heat_flow_nominal_value=1  heat_exch_flow_specify=off  heat_exch_flow_priority=High  heat_exch_flow=0 J/s  heat_exch_flow_nominal_specify=off  heat_exch_flow_nominal_unit=J/s  heat_exch_flow_nominal_value=1
  Node Potential Sensor : Subsystem
  A : PMIOPort  Port=1  Side=Left
  MAP : Outport
  MAT : Outport  Port=2
  wires:
  Node Potential Sensor/2(T (C)) -> MAT/1
  Node Potential Sensor/1(P (KPa)) -> MAP/1
  connections:
  Intake Manifold Volume1/LConn2 -- Heat-Transfer Neglected/LConn1
  A/RConn1 -- Intake Manifold Volume1/LConn1 -- Node Potential Sensor/LConn1

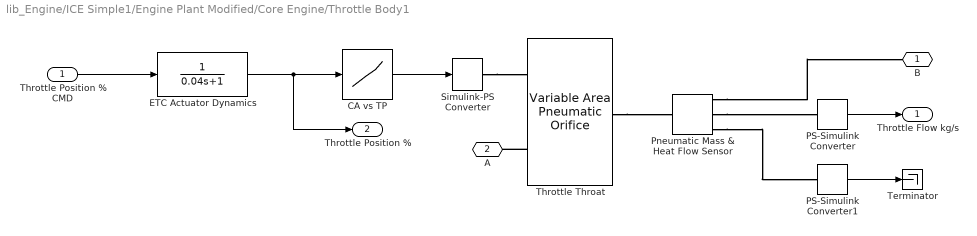
== system lib_Engine/ICE Simple1/Engine Plant Modified/Core Engine/Throttle Body1 ==
  Throttle Position % CMD : Inport
  CA vs TP : Lookup  InputValues=Engine.Throttle.CA.TPP  Table=Engine.Throttle.CA.CA  LookUpMeth=Interpolation-Use End Values
  ETC Actuator Dynamics : TransferFcn  Denominator=[0.04 1]
  PS-Simulink Converter : nesl_utility/PS-Simulink Converter  PhysicalDomain=network_engine_domain  SubClassName=ps_output  LeftPortType=input  RightPortType=output  PseudoPeriodic=off  Frequencies=[]  Unit=g/s  AffineConversion=off
  PS-Simulink Converter1 : nesl_utility/PS-Simulink Converter  PhysicalDomain=network_engine_domain  SubClassName=ps_output  LeftPortType=input  RightPortType=output  PseudoPeriodic=off  Frequencies=[]  Unit=J/s  AffineConversion=off
  Pneumatic Mass & Heat Flow Sensor : Pneumatic_lib/Pneumatic Sensors/Pneumatic Mass & Heat Flow Sensor
  Simulink-PS Converter : nesl_utility/Simulink-PS Converter  PhysicalDomain=network_engine_domain  SubClassName=ps_input  LeftPortType=input  RightPortType=output  PseudoPeriodic=off  Frequencies=[]  NoiseDistribution=none  NoiseParameters=[]  Unit=m^2  AffineConversion=off  FilteringAndDerivatives=zero  SimscapeFilterOrder=1  InputFilterTimeConstant=.001  UdotUserProvided=0
  Terminator : Terminator
  Throttle Throat : Pneumatic_lib/Pneumatic Elements/Variable Area Pneumatic Orifice  Cd=1  Area0=1e-7 m^2  G_specify=off  G_priority=High  G=0 kg/s  G_nominal_specify=off  G_nominal_unit=kg/s  G_nominal_value=1  Q1_specify=off  Q1_priority=High  Q1=0 J/s  Q1_nominal_specify=off  Q1_nominal_unit=J/s  Q1_nominal_value=1  Q2_specify=off  Q2_priority=High  Q2=0 J/s  Q2_nominal_specify=off  Q2_nominal_unit=J/s  Q2_nominal_value=1  p1_specify=off  p1_priority=High  p1=1e+5 Pa  p1_nominal_specify=off  p1_nominal_unit=Pa  p1_nominal_value=1  p2_specify=off  p2_priority=High  p2=1e+5 Pa  p2_nominal_specify=off  p2_nominal_unit=Pa  p2_nominal_value=1  T1_specify=off  T1_priority=High  T1=300 K  T1_nominal_specify=off  T1_nominal_unit=K  T1_nominal_value=1  T2_specify=off  T2_priority=High  T2=300 K  T2_nominal_specify=off  T2_nominal_unit=K  T2_nominal_value=1
  B : PMIOPort  Port=1  Side=Right
  A : PMIOPort  Port=2  Side=Left
  Throttle Flow kg/s : Outport
  Throttle Position % : Outport  Port=2
  wires:
  Throttle Position % CMD/1 -> ETC Actuator Dynamics/1
  PS-Simulink Converter1/1 -> Terminator/1
  PS-Simulink Converter/1 -> Throttle Flow kg/s/1
  CA vs TP/1 -> Simulink-PS Converter/1
  ETC Actuator Dynamics/1 -> CA vs TP/1, Throttle Position %/1
  connections:
  Pneumatic Mass & Heat Flow Sensor/RConn1 -- B/RConn1
  Throttle Throat/RConn1 -- Pneumatic Mass & Heat Flow Sensor/LConn1
  Pneumatic Mass & Heat Flow Sensor/RConn3 -- PS-Simulink Converter1/LConn1
  Pneumatic Mass & Heat Flow Sensor/RConn2 -- PS-Simulink Converter/LConn1
  Throttle Throat/LConn1 -- A/RConn1
  Simulink-PS Converter/RConn1 -- Throttle Throat/LConn2

== system lib_Engine/ICE Simple1/Engine Plant Modified/Radiator/Divide by Zero Fix ==
  Multiply : Inport
  Divide : Inport  Port=2
  Compare To Zero : simulink/Logic and Bit Operations/Compare To Zero  relop===  OutDataTypeStr=boolean
  Constant1 : Constant  Value=0
  Constant2 : Constant
  Product2 : Product  Inputs=/*  SaturateOnIntegerOverflow=on  InputSameDT=on  OutDataTypeStr=Inherit: Same as first input
  Switch : Switch  Threshold=1
  Switch1 : Switch  Threshold=1
  Output : Outport
  wires:
  Compare To Zero/1 -> Switch/2, Switch1/2
  Constant2/1 -> Switch/1
  Divide/1 -> Compare To Zero/1, Switch/3
  Switch/1 -> Product2/1
  Product2/1 -> Switch1/3
  Constant1/1 -> Switch1/1
  Switch1/1 -> Output/1
  Multiply/1 -> Product2/2

== system lib_Engine/ICE Simple1/Soft ECM/Fuel Consumption/Divide by Zero Fix ==
  Divide : Inport
  Multiply : Inport  Port=2
  Compare To Zero : simulink/Logic and Bit Operations/Compare To Zero  relop===  OutDataTypeStr=boolean
  Constant1 : Constant  Value=0
  Constant2 : Constant
  Divide1 : InportShadow
  Product2 : Product  Inputs=/*  SaturateOnIntegerOverflow=on  InputSameDT=on  OutDataTypeStr=Inherit: Same as first input
  Switch : Switch  Criteria=u2 > Threshold
  Switch1 : Switch  Criteria=u2 ~= 0
  Output : Outport
  wires:
  Divide1/1 -> Switch1/2
  Divide/1 -> Compare To Zero/1, Switch/3
  Compare To Zero/1 -> Switch/2
  Constant2/1 -> Switch/1
  Switch/1 -> Product2/1
  Product2/1 -> Switch1/1
  Constant1/1 -> Switch1/3
  Switch1/1 -> Output/1
  Multiply/1 -> Product2/2

== system lib_Engine/ICE Simple1/Soft ECM/Fuel Consumption/Divide by Zero Fix1 ==
  Divide : Inport
  Multiply : Inport  Port=2
  Compare To Zero : simulink/Logic and Bit Operations/Compare To Zero  relop===  OutDataTypeStr=boolean
  Constant1 : Constant  Value=0
  Constant2 : Constant
  Divide1 : InportShadow
  Product2 : Product  Inputs=/*  SaturateOnIntegerOverflow=on  InputSameDT=on  OutDataTypeStr=Inherit: Same as first input
  Switch : Switch  Criteria=u2 > Threshold
  Switch1 : Switch  Criteria=u2 ~= 0
  Output : Outport
  wires:
  Divide/1 -> Compare To Zero/1, Switch/3
  Product2/1 -> Switch1/1
  Constant2/1 -> Switch/1
  Switch/1 -> Product2/1
  Switch1/1 -> Output/1
  Constant1/1 -> Switch1/3
  Compare To Zero/1 -> Switch/2
  Multiply/1 -> Product2/2
  Divide1/1 -> Switch1/2

== system lib_Engine/ICE Simple1/Engine Plant Modified/Core Engine/Core Engine1/Upstream States ==
  K Converter : nesl_utility/PS-Simulink Converter  PhysicalDomain=network_engine_domain  SubClassName=ps_output  LeftPortType=input  RightPortType=output  PseudoPeriodic=off  Frequencies=[]  Unit=K  AffineConversion=off
  Pa Converter : nesl_utility/PS-Simulink Converter  PhysicalDomain=network_engine_domain  SubClassName=ps_output  LeftPortType=input  RightPortType=output  PseudoPeriodic=off  Frequencies=[]  Unit=Pa  AffineConversion=off
  Pneumatic Absolute Reference : Pneumatic_lib/Pneumatic Elements/Pneumatic Absolute Reference
  Pneumatic Pressure & Temperature Sensor : Pneumatic_lib/Pneumatic Sensors/Pneumatic Pressure & Temperature Sensor
  A : PMIOPort  Port=1  Side=Left
  P (Pa) : Outport
  T (K) : Outport  Port=2
  wires:
  K Converter/1 -> T (K)/1
  Pa Converter/1 -> P (Pa)/1
  connections:
  Pneumatic Pressure & Temperature Sensor/RConn2 -- Pa Converter/LConn1
  K Converter/LConn1 -- Pneumatic Pressure & Temperature Sensor/RConn3
  Pneumatic Pressure & Temperature Sensor/LConn1 -- A/RConn1
  Pneumatic Pressure & Temperature Sensor/RConn1 -- Pneumatic Absolute Reference/LConn1

== system lib_Engine/ICE Simple1/Engine Plant Modified/Core Engine/EngEfficiency1/Divide by Zero Fix ==
  Multiply : Inport
  Divide : Inport  Port=2
  Compare To Zero : simulink/Logic and Bit Operations/Compare To Zero  relop===  OutDataTypeStr=boolean
  Constant1 : Constant  Value=0
  Constant2 : Constant
  Product2 : Product  Inputs=/*  SaturateOnIntegerOverflow=on  InputSameDT=on  OutDataTypeStr=Inherit: Same as first input
  Switch : Switch  Threshold=1
  Switch1 : Switch  Threshold=1
  Output : Outport
  wires:
  Compare To Zero/1 -> Switch/2, Switch1/2
  Constant2/1 -> Switch/1
  Divide/1 -> Compare To Zero/1, Switch/3
  Switch/1 -> Product2/1
  Product2/1 -> Switch1/3
  Constant1/1 -> Switch1/1
  Switch1/1 -> Output/1
  Multiply/1 -> Product2/2

== system lib_Engine/ICE Simple1/Engine Plant Modified/Core Engine/Intake Manifold1/Node Potential Sensor ==
  K Converter : nesl_utility/PS-Simulink Converter  PhysicalDomain=network_engine_domain  SubClassName=ps_output  LeftPortType=input  RightPortType=output  PseudoPeriodic=off  Frequencies=[]  Unit=K  AffineConversion=off
  K to C : Fcn  Expr=u(1)-273.15
  Pa Converter : nesl_utility/PS-Simulink Converter  PhysicalDomain=network_engine_domain  SubClassName=ps_output  LeftPortType=input  RightPortType=output  PseudoPeriodic=off  Frequencies=[]  Unit=Pa  AffineConversion=off
  Pa to KPa : Gain  Gain=0.001
  Pneumatic Absolute Reference : Pneumatic_lib/Pneumatic Elements/Pneumatic Absolute Reference
  Pneumatic Pressure & Temperature Sensor : Pneumatic_lib/Pneumatic Sensors/Pneumatic Pressure & Temperature Sensor
  A : PMIOPort  Port=1  Side=Left
  P (KPa) : Outport
  T (C) : Outport  Port=2
  wires:
  Pa to KPa/1 -> P (KPa)/1
  K to C/1 -> T (C)/1
  K Converter/1 -> K to C/1
  Pa Converter/1 -> Pa to KPa/1
  connections:
  Pneumatic Pressure & Temperature Sensor/RConn2 -- Pa Converter/LConn1
  K Converter/LConn1 -- Pneumatic Pressure & Temperature Sensor/RConn3
  Pneumatic Pressure & Temperature Sensor/LConn1 -- A/RConn1
  Pneumatic Pressure & Temperature Sensor/RConn1 -- Pneumatic Absolute Reference/LConn1

== stateflow chart lib_Engine/ICE Simple1/Engine Plant Modified/Core Engine/Crank Process ==
  state Starter_Crank
    du:
    EngActTrq = function(EngSpd_RPM);
  state Eng_Off
    du:
    EngActTrq = 0;
  state Eng_Combustion
    du:
    EngActTrq = 100;
  state CrankTrq = function(EngSpd) [function]
  state Eng_Run
    du:
    EngActTrq = EngBrkTrq;
  (default) -> Eng_Off
  Eng_Off -> Starter_Crank : [EngCrankCmd]
  Starter_Crank -> Eng_Off [order 2] : [!EngCrankCmd]
  Eng_Run -> Eng_Off : [AvlblFuel <= 0.01|| EngShutdown == 1]
  Starter_Crank -> Eng_Combustion [order 1] : [AvlblFuel >= 0.1]
  Eng_Combustion -> Eng_Run : [EngRunAtv]
  data: CrankTrq function_output; EngSpd function_input; EngRunAtv input boolean; AvlblFuel input double; EngActTrq output double; EngCrankCmd input boolean; EngBrkTrq input double; EngSpd_RPM input double; EngShutdown input boolean

== stateflow chart lib_Engine/ICE Simple1/Soft ECM/ECM_RollingAliveCnt/Rolling Alive Counter ==
  state RollingAliveCounter
    state Count1
      en: RollingAliveCnt = 0;
    state Count2
      en: RollingAliveCnt = 1;
    state Count3
      en: RollingAliveCnt = 2;
    state Count4
      en: RollingAliveCnt = 3;
    (default) -> Count1
    Count4 -> Count1 : after(0.01,sec)
    Count1 -> Count2 : after(0.01,sec)
    Count2 -> Count3 : after(0.01,sec)
    Count3 -> Count4 : after(0.01,sec)
  data: RollingAliveCnt output int8 =0

== stateflow chart lib_Engine/ICE Simple1/Soft ECM/Logic ==
  state Eng_Crank
    en:
    EngCrankCmd = 1;
    FuelPumpEnable = 1;
    EngShutdown = 0;
  state Eng_Off
    en:
    EngRunAtv = 0;
    EngCrankCmd = 0;
    ThrottleCmd = 0;
    FuelPumpEnable = 0;
  state Eng_On
    en:
    EngRunAtv = 1;
    EngCrankCmd = 0;
    du:
    ThrottleCmd = APP2TP(drvAPP,EngSpd_RPM);
  state TP = APP2TP(APP,EngSpd) [function]
  (default) -> Eng_Off
  Eng_Off -> Eng_Crank : [SysPwrMd == 3]
  Eng_Crank -> Eng_Off [order 2] : [SysPwrMd < 3]
  Eng_On -> Eng_Off : [SysPwrMd < 2 || EngSpd_RPM < 500]
      | {EngShutdown = 1; }
  Eng_Crank -> Eng_On [order 1] : [EngSpd_RPM >= 580]
  data: TP function_output; APP function_input; EngSpd function_input; drvAPP input; ThrottleCmd output double; EngCrankCmd output boolean; SysPwrMd input int8; ShftLvrPos input int8; EngSpd_RPM input double; VehSpdAvgDrvn input double; EngRunAtv output boolean; FuelPumpEnable output double; EngShutdown output boolean
